simulink subsystem "Arm_Length_Calculation"  (R2023b)
settings: Solver=VariableStepAuto  StartTime=0.0  StopTime=10.0  RelTol=1e-3
libraries: Controls_Components_lib x4
settings Model: Creator=ander  LastModifiedBy=ander

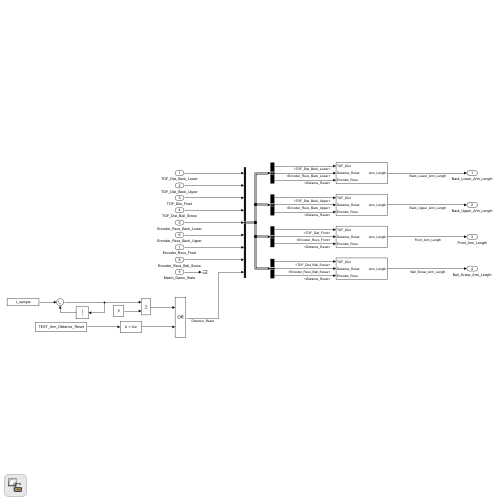
[thumbnail: Simulink's stored preview of the top-level diagram]
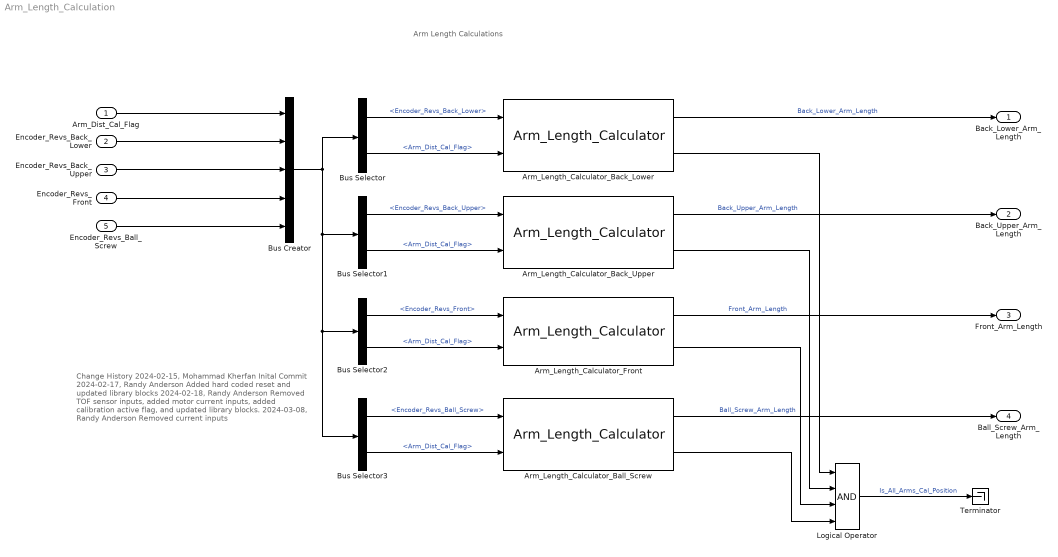
== system Arm_Length_Calculation ==
  note: Arm Length Calculations
  note: Change History
      | 2024-02-15, Mohammad Kherfan
      | Inital Commit
      | 2024-02-17, Randy Anderson
      | Added hard coded reset and updated library blocks
      | 2024-02-18, Randy Anderson
      | Removed TOF sensor inputs, added motor current inputs,
      | added calibration active flag, and updated library blocks.
      | 2024-03-08, Randy Anderson
      | Removed current inputs
  Arm_Dist_Cal_Flag : Inport
  Encoder_Revs_Back_Lower : Inport  Port=2
  Encoder_Revs_Back_Upper : Inport  Port=3
  Encoder_Revs_Front : Inport  Port=4
  Encoder_Revs_Ball_Screw : Inport  Port=5
  Arm_Length_Calculator_Back_Lower : Controls_Components_lib/Arm_Length_Calculator  Rev_2_Dist=Dist_Per_Rev_Back_Lower  Dist_Reset_Value=Dist_Reset_Value_Back_Lower  Cal_Tolerance=Dist_AA_Cal_Tol
  Arm_Length_Calculator_Back_Upper : Controls_Components_lib/Arm_Length_Calculator  Rev_2_Dist=Dist_Per_Rev_Back_Upper  Dist_Reset_Value=Dist_Reset_Value_Back_Upper  Cal_Tolerance=Dist_AA_Cal_Tol
  Arm_Length_Calculator_Ball_Screw : Controls_Components_lib/Arm_Length_Calculator  Rev_2_Dist=Dist_Per_Rev_Ball_Screw  Dist_Reset_Value=Dist_Reset_Value_Ball_Screw  Cal_Tolerance=Dist_BS_Cal_Tol
  Arm_Length_Calculator_Front : Controls_Components_lib/Arm_Length_Calculator  Rev_2_Dist=Dist_Per_Rev_Front  Dist_Reset_Value=Dist_Reset_Value_Front  Cal_Tolerance=Dist_AA_Cal_Tol
  Bus Creator : BusCreator  Inputs=5
  Bus Selector : BusSelector  OutputSignals=Encoder_Revs_Back_Lower,Arm_Dist_Cal_Flag
  Bus Selector1 : BusSelector  OutputSignals=Encoder_Revs_Back_Upper,Arm_Dist_Cal_Flag
  Bus Selector2 : BusSelector  OutputSignals=Encoder_Revs_Front,Arm_Dist_Cal_Flag
  Bus Selector3 : BusSelector  OutputSignals=Encoder_Revs_Ball_Screw,Arm_Dist_Cal_Flag
  Logical Operator : Logic  Inputs=4  AllPortsSameDT=off  OutDataTypeStr=boolean
  Terminator : Terminator
  Back_Lower_Arm_Length : Outport
  Back_Upper_Arm_Length : Outport  Port=2
  Front_Arm_Length : Outport  Port=3
  Ball_Screw_Arm_Length : Outport  Port=4
  wires:
  Bus Creator/1 -> Bus Selector1/1, Bus Selector2/1, Bus Selector3/1, Bus Selector/1
  Arm_Length_Calculator_Back_Lower/1 -> Back_Lower_Arm_Length/1  "Back_Lower_Arm_Length"
  Arm_Length_Calculator_Back_Upper/1 -> Back_Upper_Arm_Length/1  "Back_Upper_Arm_Length"
  Arm_Length_Calculator_Front/1 -> Front_Arm_Length/1  "Front_Arm_Length"
  Arm_Length_Calculator_Ball_Screw/1 -> Ball_Screw_Arm_Length/1  "Ball_Screw_Arm_Length"
  Bus Selector/1 -> Arm_Length_Calculator_Back_Lower/1  "<Encoder_Revs_Back_Lower>"
  Bus Selector/2 -> Arm_Length_Calculator_Back_Lower/2  "<Arm_Dist_Cal_Flag>"
  Bus Selector1/1 -> Arm_Length_Calculator_Back_Upper/1  "<Encoder_Revs_Back_Upper>"
  Bus Selector1/2 -> Arm_Length_Calculator_Back_Upper/2  "<Arm_Dist_Cal_Flag>"
  Bus Selector2/1 -> Arm_Length_Calculator_Front/1  "<Encoder_Revs_Front>"
  Bus Selector2/2 -> Arm_Length_Calculator_Front/2  "<Arm_Dist_Cal_Flag>"
  Bus Selector3/1 -> Arm_Length_Calculator_Ball_Screw/1  "<Encoder_Revs_Ball_Screw>"
  Bus Selector3/2 -> Arm_Length_Calculator_Ball_Screw/2  "<Arm_Dist_Cal_Flag>"
  Arm_Dist_Cal_Flag/1 -> Bus Creator/1
  Encoder_Revs_Back_Lower/1 -> Bus Creator/2
  Encoder_Revs_Back_Upper/1 -> Bus Creator/3
  Encoder_Revs_Front/1 -> Bus Creator/4
  Encoder_Revs_Ball_Screw/1 -> Bus Creator/5
  Arm_Length_Calculator_Back_Lower/2 -> Logical Operator/1
  Arm_Length_Calculator_Back_Upper/2 -> Logical Operator/2
  Arm_Length_Calculator_Front/2 -> Logical Operator/3
  Arm_Length_Calculator_Ball_Screw/2 -> Logical Operator/4
  Logical Operator/1 -> Terminator/1  "Is_All_Arms_Cal_Position"
